simulink model "GPrimer"  (Simulink 4.00)
settings: Solver=ode45  StartTime=0.0  StopTime=10.0  RelTol=1e-3
settings Model: LastModifiedBy=user

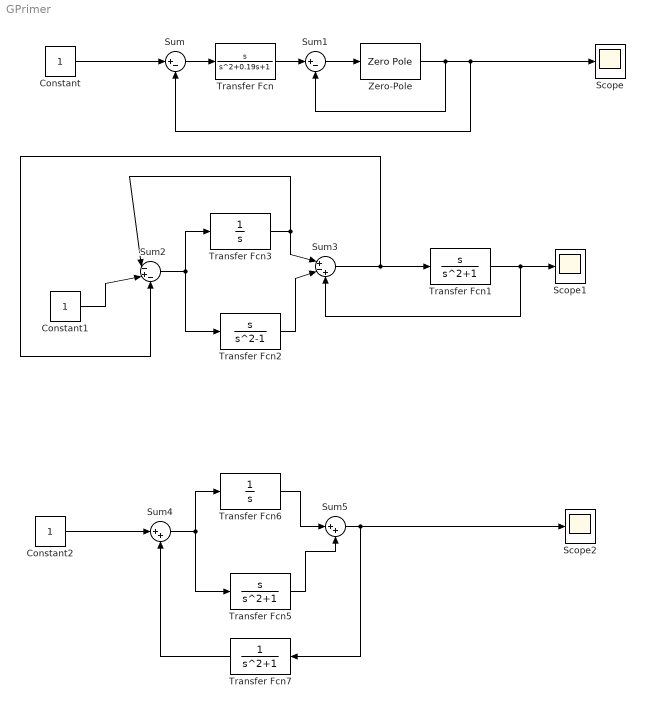
== system GPrimer ==
  Constant : Constant  Value=1
  Constant1 : Constant  Value=1
  Constant2 : Constant  Value=1
  Scope : Scope
      settings: TimeRange=20  YMin=-5  YMax=5  SaveToWorkspace=off  SaveName=ScopeData  LimitDataPoints=on  MaxDataPoints=5000
  Scope1 : Scope
      settings: TimeRange=4  YMin=-5  YMax=1  SaveToWorkspace=off  LimitDataPoints=on  MaxDataPoints=5000
  Scope2 : Scope
      settings: TimeRange=11  YMin=-5  YMax=6000  SaveToWorkspace=off  SaveName=ScopeData2  LimitDataPoints=on  MaxDataPoints=5000
  Sum : Sum  Inputs=|+-  SaturateOnIntegerOverflow=on
  Sum1 : Sum  Inputs=|+-  SaturateOnIntegerOverflow=on
  Sum2 : Sum  Inputs=|-+-  SaturateOnIntegerOverflow=on
  Sum3 : Sum  Inputs=|+-+  SaturateOnIntegerOverflow=on
  Sum4 : Sum  Inputs=|++  SaturateOnIntegerOverflow=on
  Sum5 : Sum  Inputs=|++  SaturateOnIntegerOverflow=on
  Transfer Fcn : TransferFcn  Numerator=[1 0]  Denominator=[1 0.19 1]  AbsoluteTolerance=auto  Realization=auto
  Transfer Fcn1 : TransferFcn  Numerator=[1 0]  Denominator=[1 0 1]  AbsoluteTolerance=auto  Realization=auto
  Transfer Fcn2 : TransferFcn  Numerator=[1 0]  Denominator=[1 0 -1]  AbsoluteTolerance=auto  Realization=auto
  Transfer Fcn3 : TransferFcn  Numerator=[1]  Denominator=[1 0]  AbsoluteTolerance=auto  Realization=auto
  Transfer Fcn5 : TransferFcn  Numerator=[1 0]  Denominator=[1 0 1]  AbsoluteTolerance=auto  Realization=auto
  Transfer Fcn6 : TransferFcn  Numerator=[1]  Denominator=[1 0]  AbsoluteTolerance=auto  Realization=auto
  Transfer Fcn7 : TransferFcn  Orientation=left  Numerator=[ 1]  Denominator=[1 0 1]  AbsoluteTolerance=auto  Realization=auto
  Zero-Pole : ZeroPole  Zeros=[0]  Poles=[-0.09 -1]  Gain=[1]  AbsoluteTolerance=auto
  wires:
  Sum/1 -> Transfer Fcn/1
  Transfer Fcn/1 -> Sum1/1
  Sum1/1 -> Zero-Pole/1
  Zero-Pole/1 -> Sum1/2, Sum/2, Scope/1
  Constant/1 -> Sum/1
  Constant1/1 -> Sum2/2
  Transfer Fcn3/1 -> Sum3/1, Sum2/1
  Sum3/1 -> Transfer Fcn1/1, Sum2/3
  Transfer Fcn2/1 -> Sum3/2
  Transfer Fcn1/1 -> Scope1/1, Sum3/3
  Sum2/1 -> Transfer Fcn2/1, Transfer Fcn3/1
  Constant2/1 -> Sum4/1
  Transfer Fcn6/1 -> Sum5/1
  Sum5/1 -> Scope2/1, Transfer Fcn7/1
  Transfer Fcn5/1 -> Sum5/2
  Sum4/1 -> Transfer Fcn5/1, Transfer Fcn6/1
  Transfer Fcn7/1 -> Sum4/2
